simulink model "LHC_18kW_v3"  (R2015a)
settings: Solver=ode15s  StartTime=0.0  StopTime=5e6  MaxStep=1e2  RelTol=1e-3
libraries: simCryogenics_lib x134, nesl_utility x90
(part 1 of 2)
settings Model: Creator=SK248285  LastModifiedBy=FB229602
settings SimscapeCC: SimscapeLogType=all  SimscapeLogLimitData=off

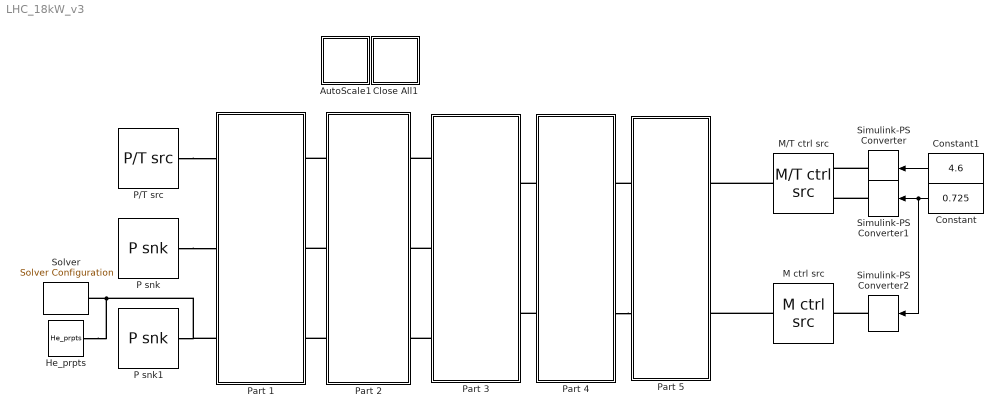
== system LHC_18kW_v3 ==
  AutoScale1 : Subsystem
      settings: OpenFcn=|
      | set(0, 'showhiddenhandles', 'on')
      | 
      | scope = findobj(0, 'Tag', 'SIMULINK_SIMSCOPE_FIGURE');
      | 
      | for i=1:length(scope)
      |   simscope('ScopeBar', 'ActionIcon', 'Find',     scope(i))
      | end
      | 
      | set(0, 'showhiddenhandles', 'off')
      mask Display: disp('Auto\nScale\nScope')
  Close All1 : Subsystem
      settings: OpenFcn=|
      | set(0, 'showhiddenhandles', 'on')
      | scope = findobj(0, 'Tag','SIMULINK_SIMSCOPE_FIGURE');
      | close(scope)
      | set(0, 'showhiddenhandles', 'off')
      mask Display: disp('Close\nAll\nScope')
  Constant : Constant  Value=0.725
  Constant1 : Constant  Value=4.6
  He_prpts : simCryogenics_lib/Utilities/He_prpts  P_min=0.1 bar  T_min=4 K  T_max=320 K  P_max=20 bar  Mol=4.0026 * 10 ^ (- 3) kg/mol
  M ctrl src : simCryogenics_lib/Sources_Sinks/M ctrl src
  M/T ctrl src : simCryogenics_lib/Sources_Sinks/M//T ctrl src
  P snk : simCryogenics_lib/Sources_Sinks/P snk  P=4 bar
  P snk1 : simCryogenics_lib/Sources_Sinks/P snk  P=1.13 bar
  P/T src : simCryogenics_lib/Sources_Sinks/P//T src  P=18.52 bar  T=302 K
  Part 1 : Subsystem
  Part 2 : Subsystem
  Part 3 : Subsystem
  Part 4 : Subsystem
  Part 5 : Subsystem
  Simulink-PS Converter : nesl_utility/Simulink-PS Converter  PhysicalDomain=network_engine_domain  SubClassName=ps_input  LeftPortType=input  RightPortType=output  PseudoPeriodic=off  Frequencies=[]  NoiseDistribution=none  NoiseParameters=[]  Unit=1  AffineConversion=off  InputFiltering=off  SimscapeFilterOrder=1  InputFilterTimeConstant=0.001  UdotUserProvided=1
  Simulink-PS Converter1 : nesl_utility/Simulink-PS Converter  PhysicalDomain=network_engine_domain  SubClassName=ps_input  LeftPortType=input  RightPortType=output  PseudoPeriodic=off  Frequencies=[]  NoiseDistribution=none  NoiseParameters=[]  Unit=1  AffineConversion=off  InputFiltering=off  SimscapeFilterOrder=1  InputFilterTimeConstant=0.001  UdotUserProvided=1
  Simulink-PS Converter2 : nesl_utility/Simulink-PS Converter  PhysicalDomain=network_engine_domain  SubClassName=ps_input  LeftPortType=input  RightPortType=output  PseudoPeriodic=off  Frequencies=[]  NoiseDistribution=none  NoiseParameters=[]  Unit=1  AffineConversion=off  InputFiltering=off  SimscapeFilterOrder=1  InputFilterTimeConstant=0.001  UdotUserProvided=1
  Solver : nesl_utility/Solver Configuration  PhysicalDomain=network_engine_domain  SubClassName=solver  LeftPortType=input  RightPortType=generic  Accelerate=off  Tones=[]  Harmonics=[]  SimulateNoise=off  Profile=off  UseLocalSampling=off  EnableSwitchedLinearOptims=on  FrequencyDomain=off  UseCCode=off  RelTol=0.001  AbsTol=1e-06  MinStep=1e-09  ToWorkspace=off  RevertToSquareIcSolve=off  NumHomotopyIterations=100  DoDC=off  ResidualTolerance=1e-09  UseLocalSolver=off  LocalSolverChoice=NE_BACKWARD_EULER_ADVANCER  LocalSolverSampleTime=5  DoFixedCost=off  MaxNonlinIter=3  MaxModeIter=2  LinearAlgebra=Sparse  DelaysMemoryBudget=1024  AutomaticFiltering=on  FilteringTimeConstant=0.001
  wires:
  Constant/1 -> Simulink-PS Converter2/1, Simulink-PS Converter1/1
  Constant1/1 -> Simulink-PS Converter/1
  connections:
  He_prpts/RConn1 -- Part 1/LConn3 -- P snk1/RConn1 -- Solver/RConn1
  Part 2/LConn1 -- Part 1/RConn1
  Part 3/LConn1 -- Part 2/RConn1
  Part 3/LConn2 -- Part 2/RConn2
  Part 2/LConn3 -- Part 1/RConn3
  Part 3/LConn3 -- Part 2/RConn3
  Part 2/LConn2 -- Part 1/RConn2
  P/T src/RConn1 -- Part 1/LConn1
  P snk/RConn1 -- Part 1/LConn2
  Part 4/LConn1 -- Part 3/RConn1
  Part 4/LConn2 -- Part 3/RConn2
  Part 5/LConn1 -- Part 4/RConn1
  Part 4/RConn2 -- Part 5/LConn2
  M/T ctrl src/RConn1 -- Part 5/RConn1
  M ctrl src/RConn1 -- Part 5/RConn2
  Simulink-PS Converter/RConn1 -- M/T ctrl src/LConn2
  Simulink-PS Converter1/RConn1 -- M/T ctrl src/LConn1
  Simulink-PS Converter2/RConn1 -- M ctrl src/LConn1

== system LHC_18kW_v3/AutoScale1 ==

== system LHC_18kW_v3/Close All1 ==

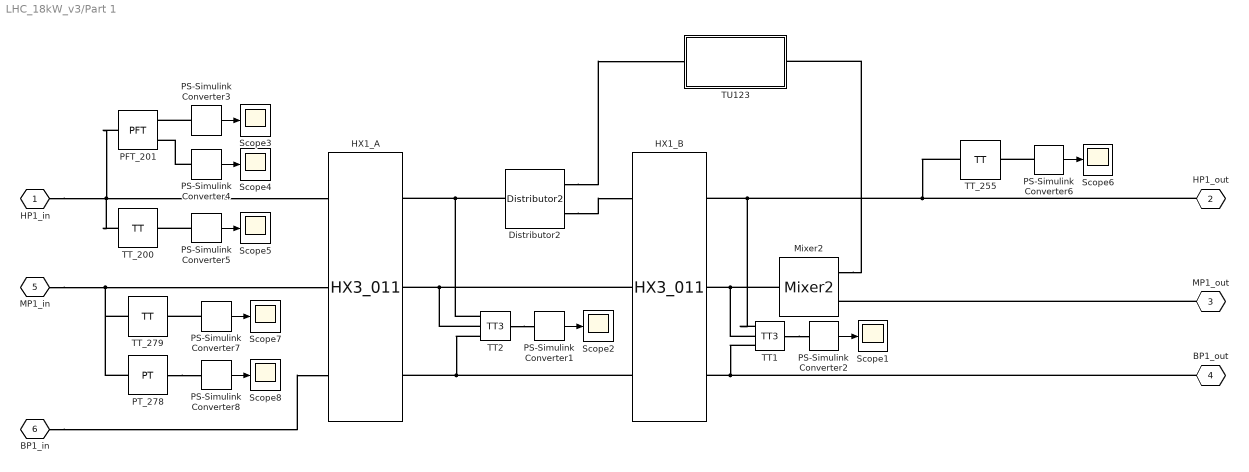
== system LHC_18kW_v3/Part 1 ==
  Distributor2 : simCryogenics_lib/Elements/Distributor2
  HX1_A : simCryogenics_lib/Elements/HX3_011  N=3  Vh=0.935 m^3  Vm=0.618 m^3  Vc=1.571 m^3  M=4593 kg  Kh=0.05 s*bar/kg  Km=0.025 s*bar/kg  Kc=0.0133 s*bar/kg  hh_m=316334 J/s/K  hh_c=316334 J/s/K  hm_c=1 J/s/K  Th0=306 K  Ph0=18.52 bar  Mh0=1.597 kg/s  Tm0=136 K  Pm0=4.07 bar  Mm0=0.8018 kg/s  Tc0=136 K  Pc0=1.05 bar  Mc0=0.7518 kg/s  sensh=0  sensm=1  sensc=1
  HX1_B : simCryogenics_lib/Elements/HX3_011  N=3  Vh=0.481 m^3  Vm=0.318 m^3  Vc=0.801 m^3  M=2366 kg  Kh=0.0586 s*bar/kg  Km=0.01247 s*bar/kg  Kc=0.0133 s*bar/kg  hh_m=119656 J/s/K  hh_c=112138 J/s/K  hm_c=1 J/s/K  Th0=143 K  Ph0=18.44 bar  Mh0=1.43 kg/s  Tm0=103 K  Pm0=4.09 bar  Mm0=0.8018 kg/s  Tc0=103 K  Pc0=1.135 bar  Mc0=0.7518 kg/s  sensh=0  sensm=1  sensc=1
  Mixer2 : simCryogenics_lib/Elements/Mixer2
  PFT_201 : simCryogenics_lib/Sensors/PFT
  PS-Simulink Converter{1..8} (8 alike) : nesl_utility/PS-Simulink Converter  PhysicalDomain=network_engine_domain  SubClassName=ps_output  LeftPortType=input  RightPortType=output  PseudoPeriodic=off  Frequencies=[]  Unit=1  AffineConversion=off
  PT_278 : simCryogenics_lib/Sensors/PT
  Scope{1..8} (8 alike) : Scope
      Scope1 settings: TimeRange=10000  SaveName=ScopeData3
      Scope2 settings: TimeRange=100000  YMin=100  YMax=400  SaveName=ScopeData11
      Scope3 settings: TimeRange=10000  SaveName=ScopeData23
      Scope4 settings: TimeRange=10000  YMin=1.89568  YMax=1.89568  SaveName=ScopeData24
      Scope5 settings: TimeRange=10000  YMin=302  YMax=302  SaveName=ScopeData38
      Scope6 settings: TimeRange=10000  SaveName=ScopeData6
      Scope7 settings: TimeRange=10000  SaveName=ScopeData39
      Scope8 settings: TimeRange=10000  SaveName=ScopeData40
  TT1 : simCryogenics_lib/Sensors/TT3
  TT2 : simCryogenics_lib/Sensors/TT3
  TT_200 : simCryogenics_lib/Sensors/TT
  TT_255 : simCryogenics_lib/Sensors/TT
  TT_279 : simCryogenics_lib/Sensors/TT
  TU123 : Subsystem
  HP1_in : PMIOPort  Port=1  Side=Left
  HP1_out : PMIOPort  Port=2  Side=Right
  MP1_out : PMIOPort  Port=3  Side=Right
  BP1_out : PMIOPort  Port=4  Side=Right
  MP1_in : PMIOPort  Port=5  Side=Left
  BP1_in : PMIOPort  Port=6  Side=Left
  wires:
  PS-Simulink Converter1/1 -> Scope2/1
  PS-Simulink Converter2/1 -> Scope1/1
  PS-Simulink Converter3/1 -> Scope3/1
  PS-Simulink Converter4/1 -> Scope4/1
  PS-Simulink Converter5/1 -> Scope5/1
  PS-Simulink Converter7/1 -> Scope7/1
  PS-Simulink Converter8/1 -> Scope8/1
  PS-Simulink Converter6/1 -> Scope6/1
  connections:
  HX1_B/LConn1 -- TT2/LConn3 -- HX1_A/RConn1
  Distributor2/LConn1 -- TT2/LConn1 -- HX1_A/RConn3
  HX1_B/LConn2 -- TT2/LConn2 -- HX1_A/RConn2
  Distributor2/RConn2 -- HX1_B/LConn3
  BP1_out/RConn1 -- TT1/LConn3 -- HX1_B/RConn1
  MP1_out/RConn1 -- Mixer2/LConn1
  Mixer2/RConn1 -- TT1/LConn2 -- HX1_B/RConn2
  HP1_in/RConn1 -- HX1_A/LConn3 -- PFT_201/LConn1 -- TT_200/LConn1
  MP1_in/RConn1 -- PT_278/LConn1 -- TT_279/LConn1 -- HX1_A/LConn2
  BP1_in/RConn1 -- HX1_A/LConn1
  HP1_out/RConn1 -- TT_255/LConn1 -- TT1/LConn1 -- HX1_B/RConn3
  Distributor2/RConn1 -- TU123/LConn1
  Mixer2/LConn2 -- TU123/RConn1
  TT2/RConn1 -- PS-Simulink Converter1/LConn1
  TT1/RConn1 -- PS-Simulink Converter2/LConn1
  PS-Simulink Converter3/LConn1 -- PFT_201/RConn1
  PS-Simulink Converter4/LConn1 -- PFT_201/RConn2
  PS-Simulink Converter5/LConn1 -- TT_200/RConn1
  PS-Simulink Converter7/LConn1 -- TT_279/RConn1
  PT_278/RConn1 -- PS-Simulink Converter8/LConn1
  PS-Simulink Converter6/LConn1 -- TT_255/RConn1

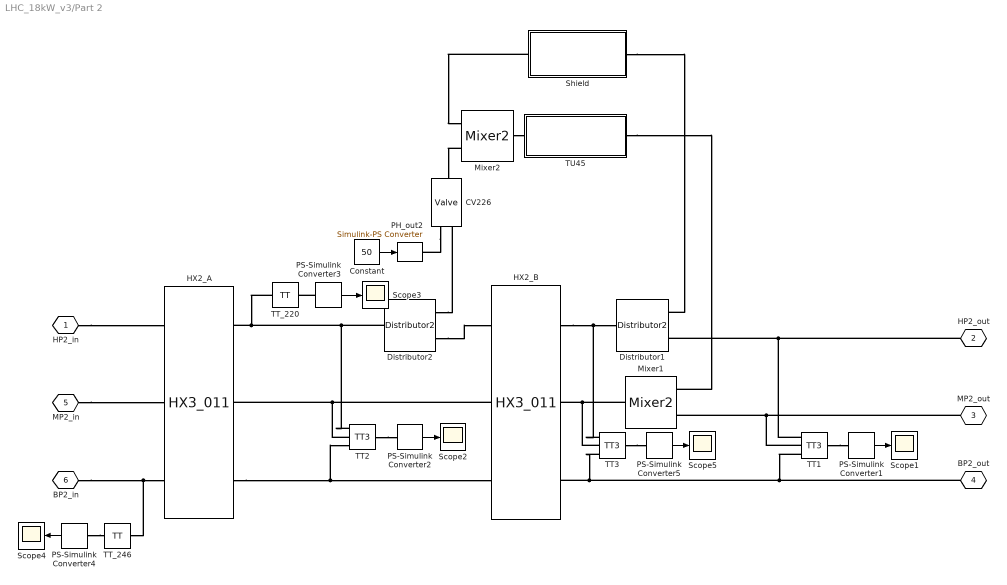
== system LHC_18kW_v3/Part 2 ==
  CV226 : simCryogenics_lib/Elements/Valve  CVmax=18.96  ControlInputMin=0  ControlInputMax=100  Xt=0.65  Rv=50  lin_v=0  lim_v=0  K=2.4e-5 m^1.50000*kg^0.50000/s/bar^0.50000  Cmd_specify=off  Cmd_priority=High  Cmd=0  gamma_specify=off  gamma_priority=High  gamma=0  rho_specify=off  rho_priority=High  rho=0 kg/m^3  Xc_specify=off  Xc_priority=High  Xc=0  X_specify=off  X_priority=High  X=0  Y_specify=off  Y_priority=High  Y=0  CV_specify=off  CV_priority=High  CV=0
  Constant : Constant  Value=50
  Distributor1 : simCryogenics_lib/Elements/Distributor2
  Distributor2 : simCryogenics_lib/Elements/Distributor2
  HX2_A : simCryogenics_lib/Elements/HX3_011  N=3  Vh=0.313 m^3  Vm=0.182 m^3  Vc=0.637 m^3  M=1697 kg  Kh=0.02198 s*bar/kg  Km=0.01754 s*bar/kg  Kc=0.01330 s*bar/kg  hh_m=111457 J/s/K  hh_c=146800 J/s/K  hm_c=1 J/s/K  Th0=94 K  Ph0=18.36 bar  Mh0=1.365 kg/s  Tm0=67 K  Pm0=4.1 bar  Mm0=0.57 kg/s  Tc0=67 K  Pc0=1.14 bar  Mc0=0.7518 kg/s  sensh=0  sensm=1  sensc=1
  HX2_B : simCryogenics_lib/Elements/HX3_011  N=3  Vh=0.344 m^3  Vm=0.182 m^3  Vc=0.637 m^3  M=1838 kg  Kh=0.02489 s*bar/kg  Km=0.01754 s*bar/kg  Kc=0.01330 s*bar/kg  hh_m=106764 J/s/K  hh_c=140360 J/s/K  hm_c=1 J/s/K  Th0=68.99 K  Ph0=18.33 bar  Mh0=1.205 kg/s  Tm0=49 K  Pm0=4.11 bar  Mm0=0.57 kg/s  Tc0=49 K  Pc0=1.15 bar  Mc0=0.7518 kg/s  sensh=0  sensm=1  sensc=1
  Mixer1 : simCryogenics_lib/Elements/Mixer2
  Mixer2 : simCryogenics_lib/Elements/Mixer2
  PH_out2 : nesl_utility/Simulink-PS Converter  PhysicalDomain=network_engine_domain  SubClassName=ps_input  LeftPortType=input  RightPortType=output  PseudoPeriodic=off  Frequencies=[]  NoiseDistribution=none  NoiseParameters=[]  Unit=bar  AffineConversion=off  InputFiltering=off  SimscapeFilterOrder=1  InputFilterTimeConstant=0.001  UdotUserProvided=1
  PS-Simulink Converter{1..5} (5 alike) : nesl_utility/PS-Simulink Converter  PhysicalDomain=network_engine_domain  SubClassName=ps_output  LeftPortType=input  RightPortType=output  PseudoPeriodic=off  Frequencies=[]  Unit=1  AffineConversion=off
  Scope{1..5} (5 alike) : Scope
      Scope1 settings: TimeRange=10000  SaveName=ScopeData17
      Scope2 settings: TimeRange=10000  SaveName=ScopeData12
      Scope3 settings: TimeRange=10000  SaveName=ScopeData10
      Scope4 settings: TimeRange=10000  SaveName=ScopeData42
      Scope5 settings: TimeRange=10000  SaveName=ScopeData65
  Shield : Subsystem
  TT1 : simCryogenics_lib/Sensors/TT3
  TT2 : simCryogenics_lib/Sensors/TT3
  TT3 : simCryogenics_lib/Sensors/TT3
  TT_220 : simCryogenics_lib/Sensors/TT
  TT_246 : simCryogenics_lib/Sensors/TT
  TU45 : Subsystem
  HP2_in : PMIOPort  Port=1  Side=Left
  HP2_out : PMIOPort  Port=2  Side=Right
  MP2_out : PMIOPort  Port=3  Side=Right
  BP2_out : PMIOPort  Port=4  Side=Right
  MP2_in : PMIOPort  Port=5  Side=Left
  BP2_in : PMIOPort  Port=6  Side=Left
  wires:
  Constant/1 -> PH_out2/1
  PS-Simulink Converter1/1 -> Scope1/1
  PS-Simulink Converter2/1 -> Scope2/1
  PS-Simulink Converter4/1 -> Scope4/1
  PS-Simulink Converter3/1 -> Scope3/1
  PS-Simulink Converter5/1 -> Scope5/1
  connections:
  Distributor2/LConn1 -- TT2/LConn1 -- TT_220/LConn1 -- HX2_A/RConn3
  Distributor2/RConn1 -- CV226/LConn2
  CV226/LConn1 -- PH_out2/RConn1
  Distributor2/RConn2 -- HX2_B/LConn3
  HX2_B/LConn2 -- TT2/LConn2 -- HX2_A/RConn2
  HX2_A/RConn1 -- TT2/LConn3 -- HX2_B/LConn1
  Mixer2/LConn2 -- CV226/RConn1
  HX2_B/RConn3 -- TT3/LConn1 -- Distributor1/LConn1
  HP2_out/RConn1 -- Distributor1/RConn2 -- TT1/LConn1
  Mixer1/RConn1 -- TT3/LConn2 -- HX2_B/RConn2
  MP2_out/RConn1 -- TT1/LConn2 -- Mixer1/LConn2
  BP2_out/RConn1 -- TT3/LConn3 -- HX2_B/RConn1 -- TT1/LConn3
  HP2_in/RConn1 -- HX2_A/LConn3
  MP2_in/RConn1 -- HX2_A/LConn2
  BP2_in/RConn1 -- TT_246/LConn1 -- HX2_A/LConn1
  Shield/RConn1 -- Mixer2/LConn1
  Shield/LConn1 -- Distributor1/RConn1
  Mixer2/RConn1 -- TU45/LConn1
  TU45/RConn1 -- Mixer1/LConn1
  TT1/RConn1 -- PS-Simulink Converter1/LConn1
  TT2/RConn1 -- PS-Simulink Converter2/LConn1
  PS-Simulink Converter4/LConn1 -- TT_246/RConn1
  PS-Simulink Converter3/LConn1 -- TT_220/RConn1
  TT3/RConn1 -- PS-Simulink Converter5/LConn1

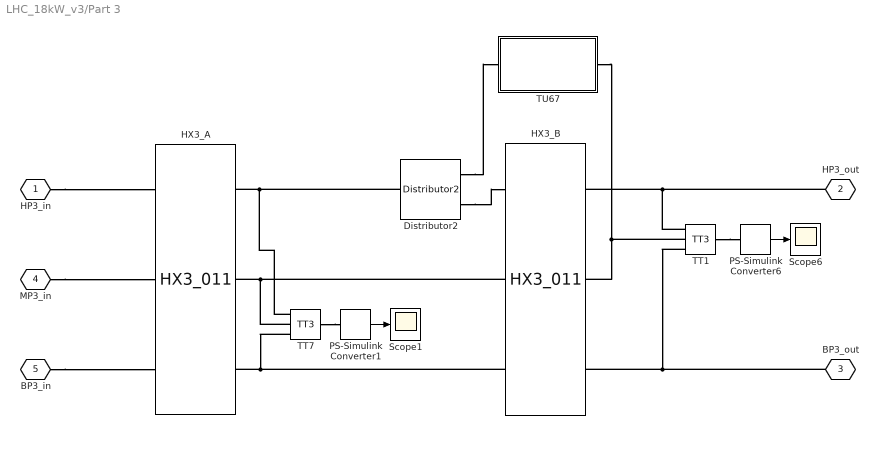
== system LHC_18kW_v3/Part 3 ==
  Distributor2 : simCryogenics_lib/Elements/Distributor2
  HX3_A : simCryogenics_lib/Elements/HX3_011  N=3  Vh=0.113 m^3  Vm=0.054 m^3  Vc=0.463 m^3  M=995 kg  Kh=0.0520 s*bar/kg  Km=0.0607 s*bar/kg  Kc=0.0133 s*bar/kg  hh_m=23169 J/s/K  hh_c=105066 J/s/K  hm_c=1 J/s/K  Th0=48 K  Ph0=18.3 bar  Mh0=0.96 kg/s  Tm0=37 K  Pm0=4.12 bar  Mm0=0.1647 kg/s  Tc0=37 K  Pc0=1.153 bar  Mc0=0.7518 kg/s  sensh=0  sensm=1  sensc=1
  HX3_B : simCryogenics_lib/Elements/HX3_011  N=3  Vh=0.135 m^3  Vm=0.06 N*m/bar  Vc=0.553 m^3  M=1188 kg  Kh=0.03143 s*bar/kg  Km=0.12143/10 s*bar/kg  Kc=0.01330 s*bar/kg  hh_m=19406 J/s/K  hh_c=128682 J/s/K  hm_c=1 J/s/K  Th0=38 K  Ph0=18.25 bar  Mh0=0.7953 kg/s  Tm0=37 K  Pm0=4.13 bar  Mm0=0.1647 kg/s  Tc0=30 K  Pc0=1.158 bar  Mc0=0.7518 kg/s  sensh=0  sensm=1  sensc=1
  PS-Simulink Converter1 : nesl_utility/PS-Simulink Converter  PhysicalDomain=network_engine_domain  SubClassName=ps_output  LeftPortType=input  RightPortType=output  PseudoPeriodic=off  Frequencies=[]  Unit=1  AffineConversion=off
  PS-Simulink Converter6 : nesl_utility/PS-Simulink Converter  PhysicalDomain=network_engine_domain  SubClassName=ps_output  LeftPortType=input  RightPortType=output  PseudoPeriodic=off  Frequencies=[]  Unit=1  AffineConversion=off
  Scope1 : Scope
      settings: TimeRange=10000  SaveName=ScopeData21
  Scope6 : Scope
      settings: TimeRange=10000  SaveName=ScopeData25
  TT1 : simCryogenics_lib/Sensors/TT3
  TT7 : simCryogenics_lib/Sensors/TT3
  TU67 : Subsystem
  HP3_in : PMIOPort  Port=1  Side=Left
  HP3_out : PMIOPort  Port=2  Side=Right
  BP3_out : PMIOPort  Port=3  Side=Right
  MP3_in : PMIOPort  Port=4  Side=Left
  BP3_in : PMIOPort  Port=5  Side=Left
  wires:
  PS-Simulink Converter1/1 -> Scope1/1
  PS-Simulink Converter6/1 -> Scope6/1
  connections:
  BP3_in/RConn1 -- HX3_A/LConn1
  MP3_in/RConn1 -- HX3_A/LConn2
  HP3_in/RConn1 -- HX3_A/LConn3
  BP3_out/RConn1 -- TT1/LConn3 -- HX3_B/RConn1
  HP3_out/RConn1 -- TT1/LConn1 -- HX3_B/RConn3
  HX3_B/LConn1 -- TT7/LConn3 -- HX3_A/RConn1
  HX3_B/LConn2 -- TT7/LConn2 -- HX3_A/RConn2
  Distributor2/RConn2 -- HX3_B/LConn3
  Distributor2/LConn1 -- TT7/LConn1 -- HX3_A/RConn3
  TU67/RConn1 -- HX3_B/RConn2 -- TT1/LConn2
  Distributor2/RConn1 -- TU67/LConn1
  TT7/RConn1 -- PS-Simulink Converter1/LConn1
  TT1/RConn1 -- PS-Simulink Converter6/LConn1

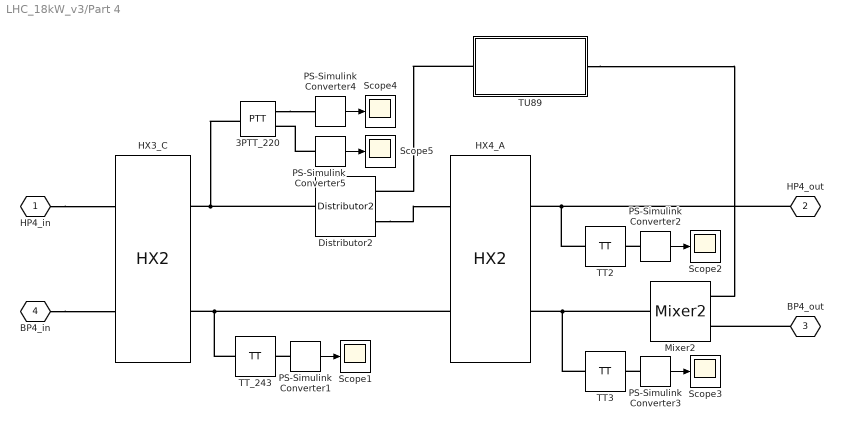
== system LHC_18kW_v3/Part 4 ==
  3PTT_220 : simCryogenics_lib/Sensors/PTT
  Distributor2 : simCryogenics_lib/Elements/Distributor2
  HX3_C : simCryogenics_lib/Elements/HX2  N=3  Vh=0.066 m^3  Vc=0.27 m^3  M=580 kg  Kh=0.0062869 s*bar/kg  Kc=0.0066507 s*bar/kg  h=66915 J/s/K  Th0=25 K  Ph0=18.225 bar  Mc0=0.7953 kg/s  Tc0=20 K  Pc0=1.16 bar  Mh0=0.7518 kg/s
  HX4_A : simCryogenics_lib/Elements/HX2  N=3  Vh=0.283 m^3  Vc=0.519 m^3  M=1821 kg  Kh=0.0121212 s*bar/kg  Kc=0.0073233 s*bar/kg  h=123127 J/s/K  Th0=21 K  Ph0=18.22 bar  Mc0=0.4125 kg/s  Tc0=9 K  Pc0=1.165 bar  Mh0=0.5462 kg/s
  Mixer2 : simCryogenics_lib/Elements/Mixer2
  PS-Simulink Converter{1..5} (5 alike) : nesl_utility/PS-Simulink Converter  PhysicalDomain=network_engine_domain  SubClassName=ps_output  LeftPortType=input  RightPortType=output  PseudoPeriodic=off  Frequencies=[]  Unit=1  AffineConversion=off
  Scope{1..5} (5 alike) : Scope
      Scope1 settings: TimeRange=10000  SaveName=ScopeData29
      Scope2 settings: TimeRange=10000  SaveName=ScopeData30
      Scope3 settings: TimeRange=10000  SaveName=ScopeData31
      Scope4 settings: TimeRange=10000  SaveName=ScopeData28
      Scope5 settings: TimeRange=10000  SaveName=ScopeData44
  TT2 : simCryogenics_lib/Sensors/TT
  TT3 : simCryogenics_lib/Sensors/TT
  TT_243 : simCryogenics_lib/Sensors/TT
  TU89 : Subsystem
  HP4_in : PMIOPort  Port=1  Side=Left
  HP4_out : PMIOPort  Port=2  Side=Right
  BP4_out : PMIOPort  Port=3  Side=Right
  BP4_in : PMIOPort  Port=4  Side=Left
  wires:
  PS-Simulink Converter1/1 -> Scope1/1
  PS-Simulink Converter2/1 -> Scope2/1
  PS-Simulink Converter3/1 -> Scope3/1
  PS-Simulink Converter4/1 -> Scope4/1
  PS-Simulink Converter5/1 -> Scope5/1
  connections:
  HP4_in/RConn1 -- HX3_C/LConn2
  BP4_in/RConn1 -- HX3_C/LConn1
  Distributor2/LConn1 -- 3PTT_220/LConn1 -- HX3_C/RConn2
  Distributor2/RConn2 -- HX4_A/LConn2
  HX4_A/LConn1 -- TT_243/LConn1 -- HX3_C/RConn1
  Mixer2/RConn1 -- TT3/LConn1 -- HX4_A/RConn1
  BP4_out/RConn1 -- Mixer2/LConn2
  HP4_out/RConn1 -- TT2/LConn1 -- HX4_A/RConn2
  PS-Simulink Converter1/LConn1 -- TT_243/RConn1
  PS-Simulink Converter2/LConn1 -- TT2/RConn1
  PS-Simulink Converter3/LConn1 -- TT3/RConn1
  TU89/LConn1 -- Distributor2/RConn1
  TU89/RConn1 -- Mixer2/LConn1
  3PTT_220/RConn1 -- PS-Simulink Converter4/LConn1
  PS-Simulink Converter5/LConn1 -- 3PTT_220/RConn2

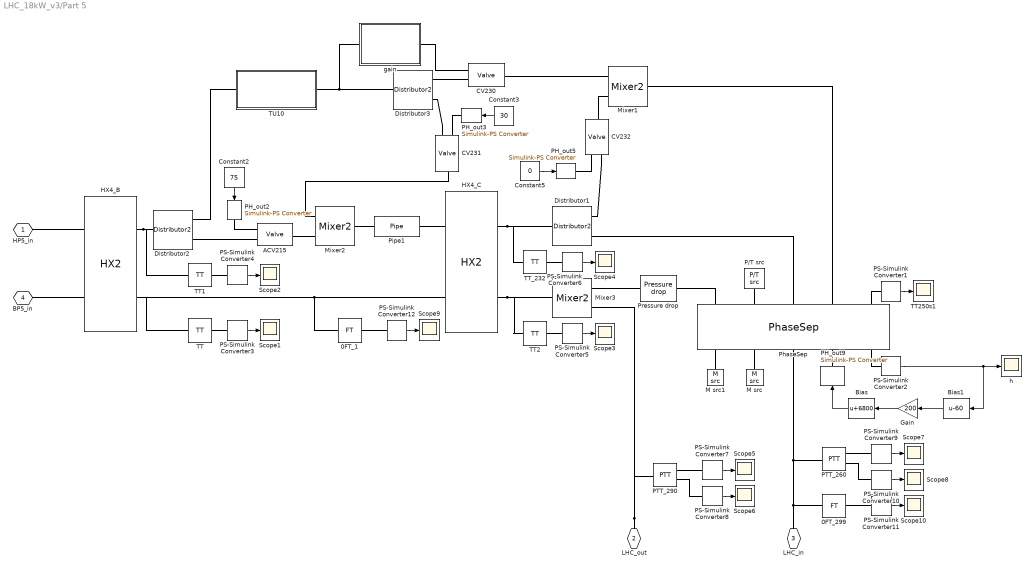
== system LHC_18kW_v3/Part 5 ==
  0FT_1 : simCryogenics_lib/Sensors/FT
  0FT_299 : simCryogenics_lib/Sensors/FT
  ACV215 : simCryogenics_lib/Elements/Valve  CVmax=8.1  ControlInputMin=0  ControlInputMax=100  Xt=0.65  Rv=50  lin_v=0  lim_v=0  K=2.4e-5 m^1.50000*kg^0.50000/s/bar^0.50000  Cmd_specify=off  Cmd_priority=High  Cmd=0  gamma_specify=off  gamma_priority=High  gamma=0  rho_specify=off  rho_priority=High  rho=0 kg/m^3  Xc_specify=off  Xc_priority=High  Xc=0  X_specify=off  X_priority=High  X=0  Y_specify=off  Y_priority=High  Y=0  CV_specify=off  CV_priority=High  CV=0
  Bias : Bias  Bias=6800
  Bias1 : Bias  Bias=-60
  CV230 : simCryogenics_lib/Elements/Valve  CVmax=8.1  ControlInputMin=0  ControlInputMax=100  Xt=0.65  Rv=50  lin_v=0  lim_v=0  K=2.4e-5 m^1.50000*kg^0.50000/s/bar^0.50000  Cmd_specify=off  Cmd_priority=High  Cmd=0  gamma_specify=off  gamma_priority=High  gamma=0  rho_specify=off  rho_priority=High  rho=0 kg/m^3  Xc_specify=off  Xc_priority=High  Xc=0  X_specify=off  X_priority=High  X=0  Y_specify=off  Y_priority=High  Y=0  CV_specify=off  CV_priority=High  CV=0
  CV231 : simCryogenics_lib/Elements/Valve  CVmax=52  ControlInputMin=0  ControlInputMax=100  Xt=0.65  Rv=50  lin_v=0  lim_v=0  K=2.4e-5 m^1.50000*kg^0.50000/s/bar^0.50000  Cmd_specify=off  Cmd_priority=High  Cmd=0  gamma_specify=off  gamma_priority=High  gamma=0  rho_specify=off  rho_priority=High  rho=0 kg/m^3  Xc_specify=off  Xc_priority=High  Xc=0  X_specify=off  X_priority=High  X=0  Y_specify=off  Y_priority=High  Y=0  CV_specify=off  CV_priority=High  CV=0
  CV232 : simCryogenics_lib/Elements/Valve  CVmax=8.1  ControlInputMin=0  ControlInputMax=100  Xt=0.65  Rv=50  lin_v=0  lim_v=0  K=2.4e-5 m^1.50000*kg^0.50000/s/bar^0.50000  Cmd_specify=off  Cmd_priority=High  Cmd=0  gamma_specify=off  gamma_priority=High  gamma=0  rho_specify=off  rho_priority=High  rho=0 kg/m^3  Xc_specify=off  Xc_priority=High  Xc=0  X_specify=off  X_priority=High  X=0  Y_specify=off  Y_priority=High  Y=0  CV_specify=off  CV_priority=High  CV=0
  Constant2 : Constant  Value=75
  Constant3 : Constant  Value=30
  Constant5 : Constant  Value=0
  Distributor1 : simCryogenics_lib/Elements/Distributor2
  Distributor2 : simCryogenics_lib/Elements/Distributor2
  Distributor3 : simCryogenics_lib/Elements/Distributor2
  Gain : Gain  Gain=200
  HX4_B : simCryogenics_lib/Elements/HX2  N=3  Vh=0.057 m^3  Vc=0.094 m^3  M=398 kg  Kh=0.03636 s*bar/kg  Kc=0.00306 s*bar/kg  h=10308 J/s/K  Th0=9 K  Ph0=18.215 bar  Mc0=0.72 kg/s  Tc0=4.6 K  Pc0=1.18 bar  Mh0=0.72 kg/s
  HX4_C : simCryogenics_lib/Elements/HX2  N=3  Vh=0.043 m^3  Vc=0.094 m^3  M=274 kg  Kh=0.04014 s*bar/kg  Kc=0.00306 s*bar/kg  h=7776 J/s/K  Th0=7 K  Ph0=3.03 bar  Mc0=0.4125 kg/s  Tc0=4.6 K  Pc0=1.19 bar  Mh0=0.72 kg/s
  M src : simCryogenics_lib/Sources_Sinks/M src  M=0 kg/s
  M src1 : simCryogenics_lib/Sources_Sinks/M src  M=0 kg/s
  Mixer1 : simCryogenics_lib/Elements/Mixer2
  Mixer2 : simCryogenics_lib/Elements/Mixer2
  Mixer3 : simCryogenics_lib/Elements/Mixer2
  P/T src : simCryogenics_lib/Sources_Sinks/P//T src  P=1 bar  T=300 K
  PH_out2 : nesl_utility/Simulink-PS Converter  PhysicalDomain=network_engine_domain  SubClassName=ps_input  LeftPortType=input  RightPortType=output  PseudoPeriodic=off  Frequencies=[]  NoiseDistribution=none  NoiseParameters=[]  Unit=bar  AffineConversion=off  InputFiltering=off  SimscapeFilterOrder=1  InputFilterTimeConstant=0.001  UdotUserProvided=1
  PH_out3 : nesl_utility/Simulink-PS Converter  PhysicalDomain=network_engine_domain  SubClassName=ps_input  LeftPortType=input  RightPortType=output  PseudoPeriodic=off  Frequencies=[]  NoiseDistribution=none  NoiseParameters=[]  Unit=bar  AffineConversion=off  InputFiltering=off  SimscapeFilterOrder=1  InputFilterTimeConstant=0.001  UdotUserProvided=1
  PH_out5 : nesl_utility/Simulink-PS Converter  PhysicalDomain=network_engine_domain  SubClassName=ps_input  LeftPortType=input  RightPortType=output  PseudoPeriodic=off  Frequencies=[]  NoiseDistribution=none  NoiseParameters=[]  Unit=bar  AffineConversion=off  InputFiltering=off  SimscapeFilterOrder=1  InputFilterTimeConstant=0.001  UdotUserProvided=1
  PH_out9 : nesl_utility/Simulink-PS Converter  PhysicalDomain=network_engine_domain  SubClassName=ps_input  LeftPortType=input  RightPortType=output  PseudoPeriodic=off  Frequencies=[]  NoiseDistribution=none  NoiseParameters=[]  Unit=1  AffineConversion=off  InputFiltering=off  SimscapeFilterOrder=1  InputFilterTimeConstant=0.001  UdotUserProvided=1
  PS-Simulink Converter{1..12} (12 alike) : nesl_utility/PS-Simulink Converter  PhysicalDomain=network_engine_domain  SubClassName=ps_output  LeftPortType=input  RightPortType=output  PseudoPeriodic=off  Frequencies=[]  Unit=1  AffineConversion=off
  PTT_260 : simCryogenics_lib/Sensors/PTT
  PTT_290 : simCryogenics_lib/Sensors/PTT
  PhaseSep : simCryogenics_lib/Elements/PhaseSep  Ideal1=1  DeltaT1=0 K  N1=10  h1=950.3318 W/K  Ideal2=1  DeltaT2=0.05 K  N2=10  h2=950.3318 W/K  hmax=2.1 m  S=0.9503 m^2  P0=1.26 bar  h0=50
  Pipe1 : simCryogenics_lib/Elements/Pipe  Vol=1 m^3  Ideal=0  P0=3.5 bar  T0=5.555 K
  Pressure drop : simCryogenics_lib/Utilities/Pressure drop  K=0.01/0.2 s*bar/kg
  Scope{1..10} (10 alike) : Scope
      Scope1 settings: TimeRange=10000  SaveName=ScopeData18
      Scope10 settings: TimeRange=10000  SaveName=ScopeData51
      Scope2 settings: TimeRange=10000  SaveName=ScopeData19
      Scope3 settings: TimeRange=10000  SaveName=ScopeData20
      Scope4 settings: TimeRange=10000  YMin=6.8375  YMax=6.855  SaveName=ScopeData22
      Scope5 settings: TimeRange=10000  SaveName=ScopeData47
      Scope6 settings: TimeRange=2111.844735963061  YMin=4.538853333333334  YMax=4.542266666666667  SaveName=ScopeData48
      Scope7 settings: TimeRange=10000  SaveName=ScopeData49
      Scope8 settings: TimeRange=10000  SaveName=ScopeData50
      Scope9 settings: TimeRange=10000  YMin=0.714834  YMax=0.714837  SaveName=ScopeData68
  TT : simCryogenics_lib/Sensors/TT
  TT1 : simCryogenics_lib/Sensors/TT
  TT2 : simCryogenics_lib/Sensors/TT
  TT250s1 : Scope
      settings: SaveName=TT1
  TT_232 : simCryogenics_lib/Sensors/TT
  TU10 : Subsystem
  gain : Subsystem
  h : Scope
      settings: TimeRange=250000  YMin=13  YMax=33  SaveName=TT
  HP5_in : PMIOPort  Port=1  Side=Left
  LHC_out : PMIOPort  Port=2  Side=Right
  LHC_in : PMIOPort  Port=3  Side=Right
  BP5_in : PMIOPort  Port=4  Side=Left
  wires:
  PS-Simulink Converter11/1 -> Scope10/1
  PS-Simulink Converter10/1 -> Scope8/1
  PS-Simulink Converter9/1 -> Scope7/1
  PS-Simulink Converter8/1 -> Scope6/1
  PS-Simulink Converter7/1 -> Scope5/1
  PS-Simulink Converter6/1 -> Scope4/1
  PS-Simulink Converter5/1 -> Scope3/1
  PS-Simulink Converter4/1 -> Scope2/1
  PS-Simulink Converter3/1 -> Scope1/1
  Bias/1 -> PH_out9/1
  PS-Simulink Converter2/1 -> Bias1/1, h/1
  PS-Simulink Converter1/1 -> TT250s1/1
  Constant5/1 -> PH_out5/1
  Constant3/1 -> PH_out3/1
  Constant2/1 -> PH_out2/1
  Bias1/1 -> Gain/1
  Gain/1 -> Bias/1
  PS-Simulink Converter12/1 -> Scope9/1
  connections:
  0FT_299/RConn1 -- PS-Simulink Converter11/LConn1
  PTT_260/RConn1 -- PS-Simulink Converter9/LConn1
  PS-Simulink Converter10/LConn1 -- PTT_260/RConn2
  PTT_290/RConn1 -- PS-Simulink Converter7/LConn1
  PS-Simulink Converter8/LConn1 -- PTT_290/RConn2
  TT_232/RConn1 -- PS-Simulink Converter6/LConn1
  TT2/RConn1 -- PS-Simulink Converter5/LConn1
  TT1/RConn1 -- PS-Simulink Converter4/LConn1
  TT/RConn1 -- PS-Simulink Converter3/LConn1
  TU10/LConn1 -- Distributor2/RConn1
  TU10/RConn1 -- Distributor3/LConn1 -- gain/LConn1
  Pressure drop/LConn1 -- PhaseSep/LConn1
  M src1/RConn1 -- PhaseSep/RConn1
  PhaseSep/RConn4 -- PH_out9/RConn1
  PS-Simulink Converter2/LConn1 -- PhaseSep/RConn5
  PS-Simulink Converter1/LConn1 -- PhaseSep/LConn5
  M src/RConn1 -- PhaseSep/RConn2
  P/T src/RConn1 -- PhaseSep/LConn2
  Distributor1/RConn2 -- PhaseSep/LConn3
  Pipe1/RConn1 -- HX4_C/LConn2
  Pipe1/LConn1 -- Mixer2/RConn1
  0FT_299/LConn1 -- PhaseSep/RConn3 -- PTT_260/LConn1 -- LHC_in/RConn1
  Pressure drop/RConn1 -- Mixer3/LConn1
  LHC_out/RConn1 -- PTT_290/LConn1 -- Mixer3/LConn2
  HX4_C/RConn1 -- TT2/LConn1 -- Mixer3/RConn1
  Mixer1/RConn1 -- PhaseSep/LConn4
  Mixer1/LConn2 -- CV232/RConn1
  CV232/LConn2 -- Distributor1/RConn1
  PH_out5/RConn1 -- CV232/LConn1
  HX4_C/RConn2 -- TT_232/LConn1 -- Distributor1/LConn1
  Mixer2/LConn1 -- CV231/RConn1
  Distributor3/RConn1 -- CV230/LConn2
  CV230/RConn1 -- Mixer1/LConn1
  PH_out3/RConn1 -- CV231/LConn1
  CV231/LConn2 -- Distributor3/RConn2
  Mixer2/LConn2 -- ACV215/RConn1
  PH_out2/RConn1 -- ACV215/LConn1
  Distributor2/RConn2 -- ACV215/LConn2
  HX4_B/LConn2 -- HP5_in/RConn1
  HX4_B/LConn1 -- BP5_in/RConn1
  TT/LConn1 -- HX4_B/RConn1 -- 0FT_1/LConn1 -- HX4_C/LConn1
  Distributor2/LConn1 -- TT1/LConn1 -- HX4_B/RConn2
  0FT_1/RConn1 -- PS-Simulink Converter12/LConn1
  gain/RConn1 -- CV230/LConn1

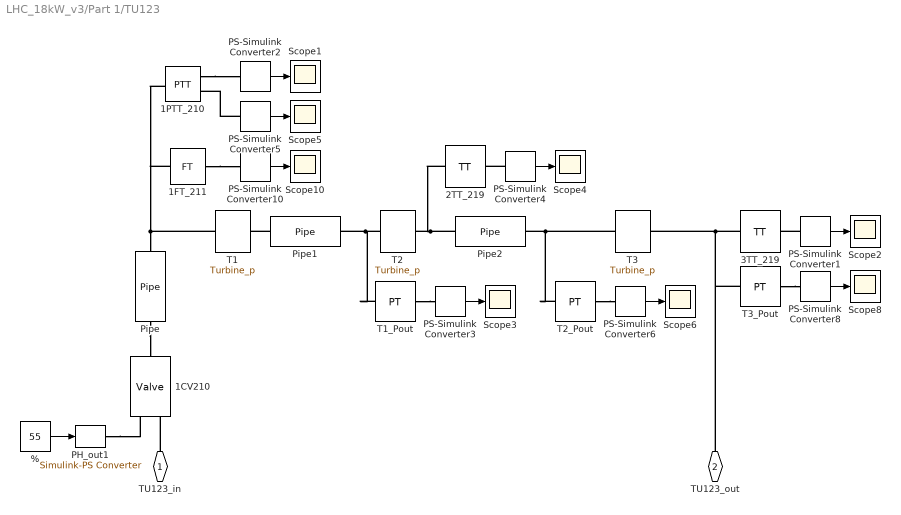
== system LHC_18kW_v3/Part 1/TU123 ==
  % : Constant  Value=55
  1CV210 : simCryogenics_lib/Elements/Valve  CVmax=26  ControlInputMin=0  ControlInputMax=100  Xt=0.65  Rv=50  lin_v=0  lim_v=0  K=2.4e-5 m^1.50000*kg^0.50000/s/bar^0.50000  Cmd_specify=off  Cmd_priority=High  Cmd=0  gamma_specify=off  gamma_priority=High  gamma=0  rho_specify=off  rho_priority=High  rho=0 kg/m^3  Xc_specify=off  Xc_priority=High  Xc=0  X_specify=off  X_priority=High  X=0  Y_specify=off  Y_priority=High  Y=0  CV_specify=off  CV_priority=High  CV=0
  1FT_211 : simCryogenics_lib/Sensors/FT
  1PTT_210 : simCryogenics_lib/Sensors/PTT
  2TT_219 : simCryogenics_lib/Sensors/TT
  3TT_219 : simCryogenics_lib/Sensors/TT
  PH_out1 : nesl_utility/Simulink-PS Converter  PhysicalDomain=network_engine_domain  SubClassName=ps_input  LeftPortType=input  RightPortType=output  PseudoPeriodic=off  Frequencies=[]  NoiseDistribution=none  NoiseParameters=[]  Unit=1  AffineConversion=off  InputFiltering=off  SimscapeFilterOrder=1  InputFilterTimeConstant=0.001  UdotUserProvided=1
  PS-Simulink Converter{1..6,8,10} (8 alike) : nesl_utility/PS-Simulink Converter  PhysicalDomain=network_engine_domain  SubClassName=ps_output  LeftPortType=input  RightPortType=output  PseudoPeriodic=off  Frequencies=[]  Unit=1  AffineConversion=off
  Pipe : simCryogenics_lib/Elements/Pipe  Vol=1 m^3  Ideal=0  P0=13 bar  T0=137 K
  Pipe1 : simCryogenics_lib/Elements/Pipe  Vol=1 m^3  Ideal=0  P0=9 bar  T0=132 K
  Pipe2 : simCryogenics_lib/Elements/Pipe  Vol=1 m^3  Ideal=0  P0=6 bar  T0=118 K
  Scope{1..6,8,10} (8 alike) : Scope
      Scope1 settings: TimeRange=10000  YMin=11.9703  YMax=11.9703  SaveName=ScopeData4
      Scope10 settings: TimeRange=10000  YMin=0.167742  YMax=0.167742
      Scope2 settings: TimeRange=10000  YMin=100  YMax=180  SaveName=ScopeData2
      Scope3 settings: TimeRange=10000  YMin=17  YMax=17.1  SaveName=ScopeData55
      Scope4 settings: TimeRange=10000  YMin=100  YMax=180  SaveName=ScopeData56
      Scope5 settings: TimeRange=10000  YMin=103.119  YMax=103.119  SaveName=ScopeData41
      Scope6 settings: TimeRange=10000  SaveName=ScopeData57
      Scope8 settings: TimeRange=10000
  T1 : simCryogenics_lib/Elements/Turbine_p  A=9.5063e-05 m^2  D=0.0296 m  Mass=1.8 kg  cst_eff=0  eta0=0.73  Tin0=137 K  Pin0=13 bar  Pout0=8.67 bar  N0=2500 1/s  Q0=0 W  v0=0  I=0 kg*m^2  gamma_specify=off  gamma_priority=High  gamma=0  C_specify=off  C_priority=High  C=0  Z_specify=off  Z_priority=High  Z=0  Cp_specify=off  Cp_priority=High  Cp=0 kJ/kg/K  Sin_specify=off  Sin_priority=High  Sin=0 kJ/kg  T_specify=off  T_priority=High  T=0 K  HoutIs_specify=off  HoutIs_priority=High  HoutIs=0 kJ/kg  u1_specify=off  u1_priority=High  u1=0 m/s  c1_specify=off  c1_priority=High  c1=0 m/s  v_specify=off  v_priority=High  v=0  eta_specify=off  eta_priority=High  eta=0  eta_var_specify=off  eta_var_priority=High  eta_var=0  N_specify=off  N_priority=High  N=0 rad/s  Q_specify=off  Q_priority=High  Q=0 W
  T1_Pout : simCryogenics_lib/Sensors/PT
  T2 : simCryogenics_lib/Elements/Turbine_p  A=1.3451e-04 m^2  D=0.0381 m  Mass=5.4 kg  cst_eff=0  eta0=0.75  Tin0=132 K  Pin0=9 bar  Pout0=6 bar  N0=1900 1/s  Q0=0 W  v0=0  I=0 kg*m^2  gamma_specify=off  gamma_priority=High  gamma=0  C_specify=off  C_priority=High  C=0  Z_specify=off  Z_priority=High  Z=0  Cp_specify=off  Cp_priority=High  Cp=0 kJ/kg/K  Sin_specify=off  Sin_priority=High  Sin=0 kJ/kg  T_specify=off  T_priority=High  T=0 K  HoutIs_specify=off  HoutIs_priority=High  HoutIs=0 kJ/kg  u1_specify=off  u1_priority=High  u1=0 m/s  c1_specify=off  c1_priority=High  c1=0 m/s  v_specify=off  v_priority=High  v=0  eta_specify=off  eta_priority=High  eta=0  eta_var_specify=off  eta_var_priority=High  eta_var=0  N_specify=off  N_priority=High  N=0 rad/s  Q_specify=off  Q_priority=High  Q=0 W
  T2_Pout : simCryogenics_lib/Sensors/PT
  T3 : simCryogenics_lib/Elements/Turbine_p  A=1.9050e-04 m^2  D=0.0471 m  Mass=5.4 kg  cst_eff=0  eta0=0.71  Tin0=118 K  Pin0=6 bar  Pout0=2.86 bar  N0=1900 1/s  Q0=0 W  v0=0  I=0 kg*m^2  gamma_specify=off  gamma_priority=High  gamma=0  C_specify=off  C_priority=High  C=0  Z_specify=off  Z_priority=High  Z=0  Cp_specify=off  Cp_priority=High  Cp=0 kJ/kg/K  Sin_specify=off  Sin_priority=High  Sin=0 kJ/kg  T_specify=off  T_priority=High  T=0 K  HoutIs_specify=off  HoutIs_priority=High  HoutIs=0 kJ/kg  u1_specify=off  u1_priority=High  u1=0 m/s  c1_specify=off  c1_priority=High  c1=0 m/s  v_specify=off  v_priority=High  v=0  eta_specify=off  eta_priority=High  eta=0  eta_var_specify=off  eta_var_priority=High  eta_var=0  N_specify=off  N_priority=High  N=0 rad/s  Q_specify=off  Q_priority=High  Q=0 W
  T3_Pout : simCryogenics_lib/Sensors/PT
  TU123_in : PMIOPort  Port=1  Side=Left
  TU123_out : PMIOPort  Port=2  Side=Right
  wires:
  %/1 -> PH_out1/1
  PS-Simulink Converter1/1 -> Scope2/1
  PS-Simulink Converter2/1 -> Scope1/1
  PS-Simulink Converter5/1 -> Scope5/1
  PS-Simulink Converter10/1 -> Scope10/1
  PS-Simulink Converter8/1 -> Scope8/1
  PS-Simulink Converter3/1 -> Scope3/1
  PS-Simulink Converter4/1 -> Scope4/1
  PS-Simulink Converter6/1 -> Scope6/1
  connections:
  TU123_in/RConn1 -- 1CV210/LConn2
  3TT_219/LConn1 -- T3_Pout/LConn1 -- TU123_out/RConn1 -- T3/RConn1
  T1/LConn1 -- 1PTT_210/LConn1 -- 1FT_211/LConn1 -- Pipe/RConn1
  Pipe/LConn1 -- 1CV210/RConn1
  PH_out1/RConn1 -- 1CV210/LConn1
  PS-Simulink Converter1/LConn1 -- 3TT_219/RConn1
  1PTT_210/RConn1 -- PS-Simulink Converter2/LConn1
  PS-Simulink Converter5/LConn1 -- 1PTT_210/RConn2
  1FT_211/RConn1 -- PS-Simulink Converter10/LConn1
  T3_Pout/RConn1 -- PS-Simulink Converter8/LConn1
  Pipe1/LConn1 -- T1/RConn1
  T2/LConn1 -- T1_Pout/LConn1 -- Pipe1/RConn1
  Pipe2/LConn1 -- 2TT_219/LConn1 -- T2/RConn1
  T3/LConn1 -- T2_Pout/LConn1 -- Pipe2/RConn1
  T1_Pout/RConn1 -- PS-Simulink Converter3/LConn1
  PS-Simulink Converter4/LConn1 -- 2TT_219/RConn1
  T2_Pout/RConn1 -- PS-Simulink Converter6/LConn1

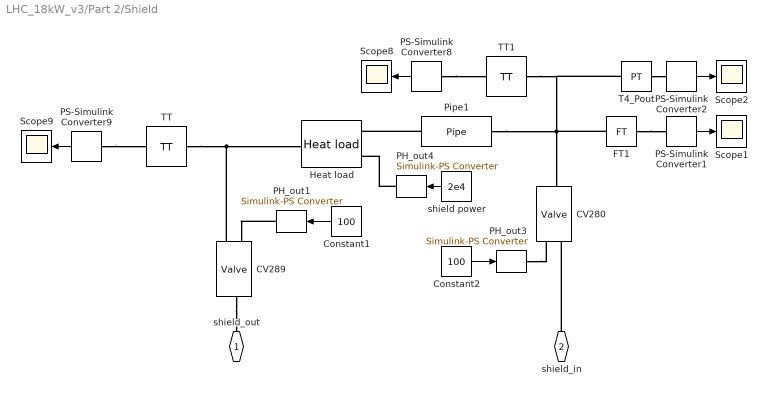
== system LHC_18kW_v3/Part 2/Shield ==
  CV280 : simCryogenics_lib/Elements/Valve  CVmax=63  ControlInputMin=0  ControlInputMax=100  Xt=0.65  Rv=50  lin_v=0  lim_v=0  K=2.4e-5 m^1.50000*kg^0.50000/s/bar^0.50000  Cmd_specify=off  Cmd_priority=High  Cmd=0  gamma_specify=off  gamma_priority=High  gamma=0  rho_specify=off  rho_priority=High  rho=0 kg/m^3  Xc_specify=off  Xc_priority=High  Xc=0  X_specify=off  X_priority=High  X=0  Y_specify=off  Y_priority=High  Y=0  CV_specify=off  CV_priority=High  CV=0
  CV289 : simCryogenics_lib/Elements/Valve  CVmax=113  ControlInputMin=0  ControlInputMax=100  Xt=0.65  Rv=50  lin_v=0  lim_v=0  K=2.4e-5 m^1.50000*kg^0.50000/s/bar^0.50000  Cmd_specify=off  Cmd_priority=High  Cmd=0  gamma_specify=off  gamma_priority=High  gamma=0  rho_specify=off  rho_priority=High  rho=0 kg/m^3  Xc_specify=off  Xc_priority=High  Xc=0  X_specify=off  X_priority=High  X=0  Y_specify=off  Y_priority=High  Y=0  CV_specify=off  CV_priority=High  CV=0
  Constant1 : Constant  Value=100
  Constant2 : Constant  Value=100
  FT1 : simCryogenics_lib/Sensors/FT
  Heat load : simCryogenics_lib/Utilities/Heat load
  PH_out1 : nesl_utility/Simulink-PS Converter  PhysicalDomain=network_engine_domain  SubClassName=ps_input  LeftPortType=input  RightPortType=output  PseudoPeriodic=off  Frequencies=[]  NoiseDistribution=none  NoiseParameters=[]  Unit=bar  AffineConversion=off  InputFiltering=off  SimscapeFilterOrder=1  InputFilterTimeConstant=0.001  UdotUserProvided=1
  PH_out3 : nesl_utility/Simulink-PS Converter  PhysicalDomain=network_engine_domain  SubClassName=ps_input  LeftPortType=input  RightPortType=output  PseudoPeriodic=off  Frequencies=[]  NoiseDistribution=none  NoiseParameters=[]  Unit=bar  AffineConversion=off  InputFiltering=off  SimscapeFilterOrder=1  InputFilterTimeConstant=0.001  UdotUserProvided=1
  PH_out4 : nesl_utility/Simulink-PS Converter  PhysicalDomain=network_engine_domain  SubClassName=ps_input  LeftPortType=input  RightPortType=output  PseudoPeriodic=off  Frequencies=[]  NoiseDistribution=none  NoiseParameters=[]  Unit=J/s  AffineConversion=off  InputFiltering=off  SimscapeFilterOrder=1  InputFilterTimeConstant=0.001  UdotUserProvided=1
  PS-Simulink Converter{1..2,8..9} (4 alike) : nesl_utility/PS-Simulink Converter  PhysicalDomain=network_engine_domain  SubClassName=ps_output  LeftPortType=input  RightPortType=output  PseudoPeriodic=off  Frequencies=[]  Unit=1  AffineConversion=off
  Pipe1 : simCryogenics_lib/Elements/Pipe  Vol=1 m^3  Ideal=0  P0=18.4 bar  T0=90 K
  Scope{1..2,8..9} (4 alike) : Scope
      Scope1 settings: TimeRange=10000  SaveName=ScopeData8
      Scope2 settings: TimeRange=10000  SaveName=ScopeData66
      Scope8 settings: TimeRange=10000  SaveName=ScopeData14
      Scope9 settings: TimeRange=10000  SaveName=ScopeData15
  T4_Pout : simCryogenics_lib/Sensors/PT
  TT : simCryogenics_lib/Sensors/TT
  TT1 : simCryogenics_lib/Sensors/TT
  shield power : Constant  Value=2e4
  shield_out : PMIOPort  Port=1  Side=Right
  shield_in : PMIOPort  Port=2  Side=Left
  wires:
  Constant1/1 -> PH_out1/1
  Constant2/1 -> PH_out3/1
  shield power/1 -> PH_out4/1
  PS-Simulink Converter1/1 -> Scope1/1
  PS-Simulink Converter8/1 -> Scope8/1
  PS-Simulink Converter9/1 -> Scope9/1
  PS-Simulink Converter2/1 -> Scope2/1
  connections:
  CV289/RConn1 -- shield_out/RConn1
  PH_out1/RConn1 -- CV289/LConn1
  CV289/LConn2 -- TT/LConn1 -- Heat load/RConn1
  Pipe1/LConn1 -- FT1/LConn1 -- CV280/RConn1 -- TT1/LConn1 -- T4_Pout/LConn1
  PH_out3/RConn1 -- CV280/LConn1
  shield_in/RConn1 -- CV280/LConn2
  PH_out4/RConn1 -- Heat load/LConn2
  Pipe1/RConn1 -- Heat load/LConn1
  FT1/RConn1 -- PS-Simulink Converter1/LConn1
  PS-Simulink Converter8/LConn1 -- TT1/RConn1
  PS-Simulink Converter9/LConn1 -- TT/RConn1
  T4_Pout/RConn1 -- PS-Simulink Converter2/LConn1

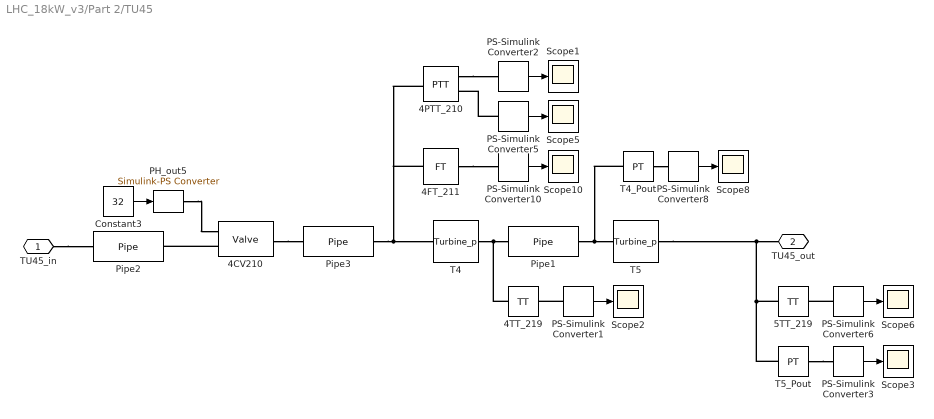
== system LHC_18kW_v3/Part 2/TU45 ==
  4CV210 : simCryogenics_lib/Elements/Valve  CVmax=75  ControlInputMin=0  ControlInputMax=100  Xt=0.65  Rv=50  lin_v=0  lim_v=0  K=2.4e-5 m^1.50000*kg^0.50000/s/bar^0.50000  Cmd_specify=off  Cmd_priority=High  Cmd=0  gamma_specify=off  gamma_priority=High  gamma=0  rho_specify=off  rho_priority=High  rho=0 kg/m^3  Xc_specify=off  Xc_priority=High  Xc=0  X_specify=off  X_priority=High  X=0  Y_specify=off  Y_priority=High  Y=0  CV_specify=off  CV_priority=High  CV=0
  4FT_211 : simCryogenics_lib/Sensors/FT
  4PTT_210 : simCryogenics_lib/Sensors/PTT
  4TT_219 : simCryogenics_lib/Sensors/TT
  5TT_219 : simCryogenics_lib/Sensors/TT
  Constant3 : Constant  Value=32
  PH_out5 : nesl_utility/Simulink-PS Converter  PhysicalDomain=network_engine_domain  SubClassName=ps_input  LeftPortType=input  RightPortType=output  PseudoPeriodic=off  Frequencies=[]  NoiseDistribution=none  NoiseParameters=[]  Unit=bar  AffineConversion=off  InputFiltering=off  SimscapeFilterOrder=1  InputFilterTimeConstant=0.001  UdotUserProvided=1
  PS-Simulink Converter{1..3,5..6,8,10} (7 alike) : nesl_utility/PS-Simulink Converter  PhysicalDomain=network_engine_domain  SubClassName=ps_output  LeftPortType=input  RightPortType=output  PseudoPeriodic=off  Frequencies=[]  Unit=1  AffineConversion=off
  Pipe1 : simCryogenics_lib/Elements/Pipe  Vol=1 m^3  Ideal=0  P0=7 bar  T0=64 K
  Pipe2 : simCryogenics_lib/Elements/Pipe  Vol=1 m^3  Ideal=0  P0=16 bar  T0=74 K
  Pipe3 : simCryogenics_lib/Elements/Pipe  Vol=1 m^3  Ideal=0  P0=11.5 bar  T0=74 K
  Scope{1..3,5..6,8,10} (7 alike) : Scope
      Scope1 settings: TimeRange=10000  YMin=10.9253  YMax=12.0753  SaveName=ScopeData7
      Scope10 settings: TimeRange=10000  YMin=0.3245  YMax=0.326  SaveName=ScopeData9
      Scope2 settings: TimeRange=10000  SaveName=ScopeData58
      Scope3 settings: TimeRange=10000  SaveName=ScopeData60
      Scope5 settings: TimeRange=10000  YMin=57.5379  YMax=57.5379  SaveName=ScopeData16
      Scope6 settings: TimeRange=10000  SaveName=ScopeData35
      Scope8 settings: TimeRange=10000  SaveName=ScopeData59
  T4 : simCryogenics_lib/Elements/Turbine_p  A=1.2806e-04 m^2  D=0.0327 m  Mass=5.4 kg  cst_eff=0  eta0=0.79  Tin0=74 K  Pin0=11.2 bar  Pout0=7 bar  N0=1780 1/s  Q0=0 W  v0=0  I=0 kg*m^2  gamma_specify=off  gamma_priority=High  gamma=0  C_specify=off  C_priority=High  C=0  Z_specify=off  Z_priority=High  Z=0  Cp_specify=off  Cp_priority=High  Cp=0 kJ/kg/K  Sin_specify=off  Sin_priority=High  Sin=0 kJ/kg  T_specify=off  T_priority=High  T=0 K  HoutIs_specify=off  HoutIs_priority=High  HoutIs=0 kJ/kg  u1_specify=off  u1_priority=High  u1=0 m/s  c1_specify=off  c1_priority=High  c1=0 m/s  v_specify=off  v_priority=High  v=0  eta_specify=off  eta_priority=High  eta=0  eta_var_specify=off  eta_var_priority=High  eta_var=0  N_specify=off  N_priority=High  N=0 rad/s  Q_specify=off  Q_priority=High  Q=0 W
  T4_Pout : simCryogenics_lib/Sensors/PT
  T5 : simCryogenics_lib/Elements/Turbine_p  A=1.8991e-04 m^2  D=0.037 m  Mass=5.4 kg  cst_eff=0  eta0=0.79  Tin0=64 K  Pin0=7 bar  Pout0=2.92 bar  N0=1900 1/s  Q0=0 W  v0=0  I=0 kg*m^2  gamma_specify=off  gamma_priority=High  gamma=0  C_specify=off  C_priority=High  C=0  Z_specify=off  Z_priority=High  Z=0  Cp_specify=off  Cp_priority=High  Cp=0 kJ/kg/K  Sin_specify=off  Sin_priority=High  Sin=0 kJ/kg  T_specify=off  T_priority=High  T=0 K  HoutIs_specify=off  HoutIs_priority=High  HoutIs=0 kJ/kg  u1_specify=off  u1_priority=High  u1=0 m/s  c1_specify=off  c1_priority=High  c1=0 m/s  v_specify=off  v_priority=High  v=0  eta_specify=off  eta_priority=High  eta=0  eta_var_specify=off  eta_var_priority=High  eta_var=0  N_specify=off  N_priority=High  N=0 rad/s  Q_specify=off  Q_priority=High  Q=0 W
  T5_Pout : simCryogenics_lib/Sensors/PT
  TU45_in : PMIOPort  Port=1  Side=Left
  TU45_out : PMIOPort  Port=2  Side=Right
  wires:
  Constant3/1 -> PH_out5/1
  PS-Simulink Converter5/1 -> Scope5/1
  PS-Simulink Converter10/1 -> Scope10/1
  PS-Simulink Converter6/1 -> Scope6/1
  PS-Simulink Converter2/1 -> Scope1/1
  PS-Simulink Converter1/1 -> Scope2/1
  PS-Simulink Converter8/1 -> Scope8/1
  PS-Simulink Converter3/1 -> Scope3/1
  connections:
  4CV210/RConn1 -- Pipe3/LConn1
  PH_out5/RConn1 -- 4CV210/LConn1
  Pipe3/RConn1 -- 4FT_211/LConn1 -- 4PTT_210/LConn1 -- T4/LConn1
  4TT_219/LConn1 -- T4/RConn1 -- Pipe1/LConn1
  TU45_in/RConn1 -- Pipe2/LConn1
  4CV210/LConn2 -- Pipe2/RConn1
  4FT_211/RConn1 -- PS-Simulink Converter10/LConn1
  PS-Simulink Converter5/LConn1 -- 4PTT_210/RConn2
  PS-Simulink Converter6/LConn1 -- 5TT_219/RConn1
  4PTT_210/RConn1 -- PS-Simulink Converter2/LConn1
  5TT_219/LConn1 -- T5/RConn1 -- TU45_out/RConn1 -- T5_Pout/LConn1
  T4_Pout/LConn1 -- Pipe1/RConn1 -- T5/LConn1
  PS-Simulink Converter1/LConn1 -- 4TT_219/RConn1
  T4_Pout/RConn1 -- PS-Simulink Converter8/LConn1
  T5_Pout/RConn1 -- PS-Simulink Converter3/LConn1

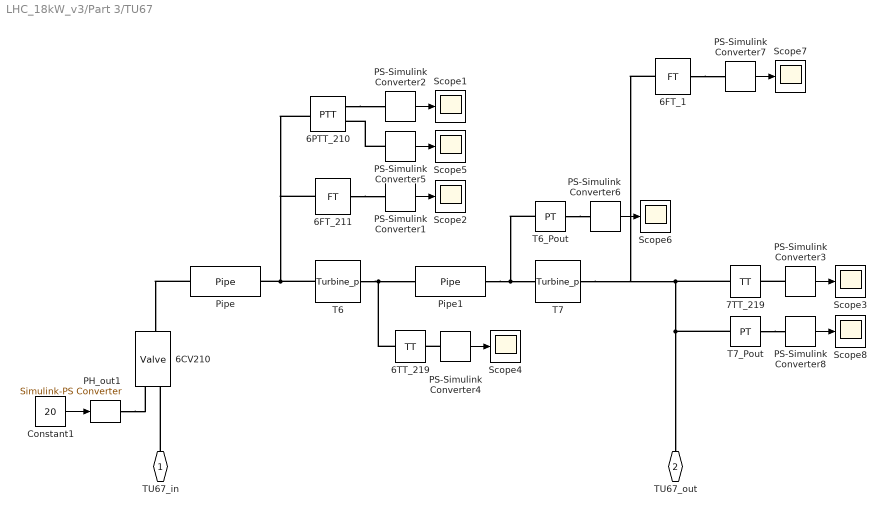
== system LHC_18kW_v3/Part 3/TU67 ==
  6CV210 : simCryogenics_lib/Elements/Valve  CVmax=58  ControlInputMin=0  ControlInputMax=100  Xt=0.65  Rv=50  lin_v=0  lim_v=0  K=2.4e-5 m^1.50000*kg^0.50000/s/bar^0.50000  Cmd_specify=off  Cmd_priority=High  Cmd=0  gamma_specify=off  gamma_priority=High  gamma=0  rho_specify=off  rho_priority=High  rho=0 kg/m^3  Xc_specify=off  Xc_priority=High  Xc=0  X_specify=off  X_priority=High  X=0  Y_specify=off  Y_priority=High  Y=0  CV_specify=off  CV_priority=High  CV=0
  6FT_1 : simCryogenics_lib/Sensors/FT
  6FT_211 : simCryogenics_lib/Sensors/FT
  6PTT_210 : simCryogenics_lib/Sensors/PTT
  6TT_219 : simCryogenics_lib/Sensors/TT
  7TT_219 : simCryogenics_lib/Sensors/TT
  Constant1 : Constant  Value=20
  PH_out1 : nesl_utility/Simulink-PS Converter  PhysicalDomain=network_engine_domain  SubClassName=ps_input  LeftPortType=input  RightPortType=output  PseudoPeriodic=off  Frequencies=[]  NoiseDistribution=none  NoiseParameters=[]  Unit=bar  AffineConversion=off  InputFiltering=off  SimscapeFilterOrder=1  InputFilterTimeConstant=0.001  UdotUserProvided=1
  PS-Simulink Converter{1..8} (8 alike) : nesl_utility/PS-Simulink Converter  PhysicalDomain=network_engine_domain  SubClassName=ps_output  LeftPortType=input  RightPortType=output  PseudoPeriodic=off  Frequencies=[]  Unit=1  AffineConversion=off
  Pipe : simCryogenics_lib/Elements/Pipe  Vol=1 m^3  Ideal=0  P0=13.5 bar  T0=37.3 K
  Pipe1 : simCryogenics_lib/Elements/Pipe  Vol=1 m^3  Ideal=0  P0=7.2 bar  T0=31.5 K
  Scope{1..8} (8 alike) : Scope
      Scope1 settings: TimeRange=10000  YMin=12.575  YMax=12.8  SaveName=ScopeData36
      Scope2 settings: TimeRange=10000  YMin=0  YMax=1  SaveName=ScopeData37
      Scope3 settings: TimeRange=10000  YMin=100  YMax=180  SaveName=ScopeData26
      Scope4 settings: TimeRange=10000  YMin=100  YMax=180  SaveName=ScopeData61
      Scope5 settings: TimeRange=10000  YMin=39.6874  YMax=39.6874  SaveName=ScopeData43
      Scope6 settings: TimeRange=10000  SaveName=ScopeData62
      Scope7 settings: TimeRange=10000  YMin=0.125559  YMax=0.125562  SaveName=ScopeData67
      Scope8 settings: TimeRange=10000  SaveName=ScopeData27
  T6 : simCryogenics_lib/Elements/Turbine_p  A=3.5404e-05 m^2  D=0.0165 m  Mass=0.6 kg  cst_eff=0  eta0=0.74  Tin0=37.3 K  Pin0=12.9 bar  Pout0=7.17 bar  N0=2780 1/s  Q0=0 W  v0=0  I=0 kg*m^2  gamma_specify=off  gamma_priority=High  gamma=0  C_specify=off  C_priority=High  C=0  Z_specify=off  Z_priority=High  Z=0  Cp_specify=off  Cp_priority=High  Cp=0 kJ/kg/K  Sin_specify=off  Sin_priority=High  Sin=0 kJ/kg  T_specify=off  T_priority=High  T=0 K  HoutIs_specify=off  HoutIs_priority=High  HoutIs=0 kJ/kg  u1_specify=off  u1_priority=High  u1=0 m/s  c1_specify=off  c1_priority=High  c1=0 m/s  v_specify=off  v_priority=High  v=0  eta_specify=off  eta_priority=High  eta=0  eta_var_specify=off  eta_var_priority=High  eta_var=0  N_specify=off  N_priority=High  N=0 rad/s  Q_specify=off  Q_priority=High  Q=0 W
  T6_Pout : simCryogenics_lib/Sensors/PT
  T7 : simCryogenics_lib/Elements/Turbine_p  A=5.7857e-05 m^2  D=0.0209 m  Mass=1.8 kg  cst_eff=0  eta0=0.76  Tin0=31.5 K  Pin0=7.2 bar  Pout0=2.94 bar  N0=2400 1/s  Q0=0 W  v0=0  I=0 kg*m^2  gamma_specify=off  gamma_priority=High  gamma=0  C_specify=off  C_priority=High  C=0  Z_specify=off  Z_priority=High  Z=0  Cp_specify=off  Cp_priority=High  Cp=0 kJ/kg/K  Sin_specify=off  Sin_priority=High  Sin=0 kJ/kg  T_specify=off  T_priority=High  T=0 K  HoutIs_specify=off  HoutIs_priority=High  HoutIs=0 kJ/kg  u1_specify=off  u1_priority=High  u1=0 m/s  c1_specify=off  c1_priority=High  c1=0 m/s  v_specify=off  v_priority=High  v=0  eta_specify=off  eta_priority=High  eta=0  eta_var_specify=off  eta_var_priority=High  eta_var=0  N_specify=off  N_priority=High  N=0 rad/s  Q_specify=off  Q_priority=High  Q=0 W
  T7_Pout : simCryogenics_lib/Sensors/PT
  TU67_in : PMIOPort  Port=1  Side=Left
  TU67_out : PMIOPort  Port=2  Side=Right
  wires:
  Constant1/1 -> PH_out1/1
  PS-Simulink Converter5/1 -> Scope5/1
  PS-Simulink Converter1/1 -> Scope2/1
  PS-Simulink Converter3/1 -> Scope3/1
  PS-Simulink Converter8/1 -> Scope8/1
  PS-Simulink Converter2/1 -> Scope1/1
  PS-Simulink Converter4/1 -> Scope4/1
  PS-Simulink Converter6/1 -> Scope6/1
  PS-Simulink Converter7/1 -> Scope7/1
  connections:
  TU67_in/RConn1 -- 6CV210/LConn2
  PH_out1/RConn1 -- 6CV210/LConn1
  Pipe/LConn1 -- 6CV210/RConn1
  T6/LConn1 -- 6FT_211/LConn1 -- 6PTT_210/LConn1 -- Pipe/RConn1
  7TT_219/LConn1 -- 6FT_1/LConn1 -- T7/RConn1 -- TU67_out/RConn1 -- T7_Pout/LConn1
  6FT_211/RConn1 -- PS-Simulink Converter1/LConn1
  PS-Simulink Converter5/LConn1 -- 6PTT_210/RConn2
  6PTT_210/RConn1 -- PS-Simulink Converter2/LConn1
  T7_Pout/RConn1 -- PS-Simulink Converter8/LConn1
  PS-Simulink Converter3/LConn1 -- 7TT_219/RConn1
  T6/RConn1 -- 6TT_219/LConn1 -- Pipe1/LConn1
  Pipe1/RConn1 -- T6_Pout/LConn1 -- T7/LConn1
  PS-Simulink Converter4/LConn1 -- 6TT_219/RConn1
  T6_Pout/RConn1 -- PS-Simulink Converter6/LConn1
  6FT_1/RConn1 -- PS-Simulink Converter7/LConn1
